simulink model "SimClassic"  (R2017a)
settings: Solver=FixedStepAuto  StartTime=0.0  StopTime=time(end)  FixedStep=0.1  RelTol=1e-3
PostLoadFcn:
  | load Classic_data_2017-11-06_16-06.mat
  | load Trajectory_data_Cux_Visby.rtz2017-11-16_14-55.mat
undefined symbols (not defined in the file): D_psi, D_u, I_psi, I_u, P_psi, P_u, toMpS, toRad, toRPS
settings Model: Creator=c00rts11  LastModifiedBy=c00rts11
settings SolverCC: ZeroCrossAlgorithm=Adaptive

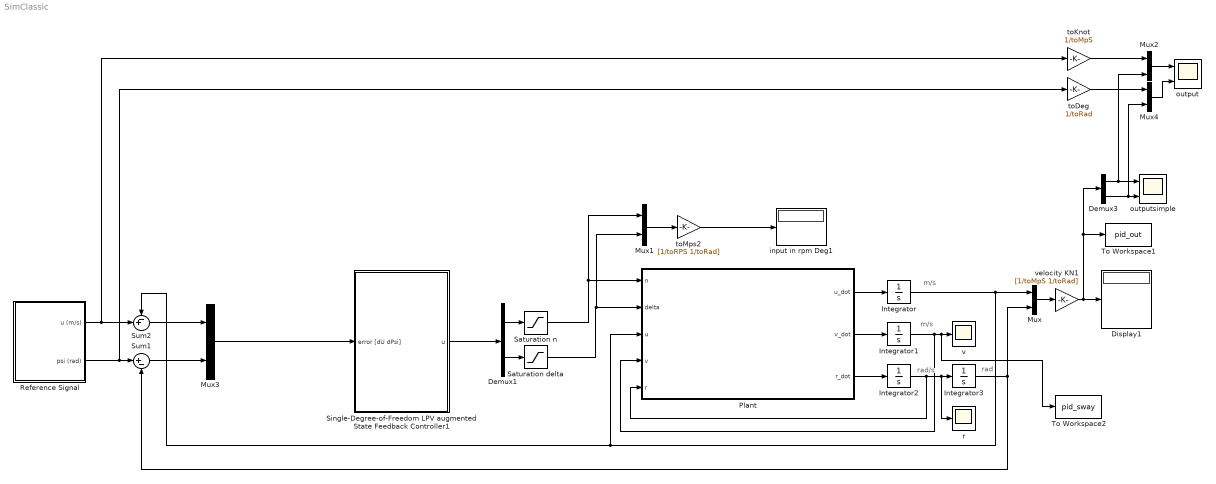
== system SimClassic ==
  note: rad
  note: rad/s
  note: m/s
  note: m/s
  Demux1 : Demux  Outputs=2
  Demux3 : Demux  Outputs=2
  Display1 : Display
  Integrator : Integrator  InitialCondition=0.1*toMpS  UpperSaturationLimit=16*toMpS  LowerSaturationLimit=1e-1*toMpS
  Integrator1 : Integrator  UpperSaturationLimit=0*toMpS  LowerSaturationLimit=-0.001*toMpS
  Integrator2 : Integrator
  Integrator3 : Integrator  WrapState=on  WrappedStateUpperValue=180*toRad  WrappedStateLowerValue=-180*toRad
  Mux{,1..4} (5 alike) : Mux  Inputs=2
  Plant : MATLAB Function  TreatAsAtomicUnit=on
  Reference Signal : Subsystem
  Saturation delta : Saturate  UpperLimit=30*toRad  LowerLimit=-30*toRad  LinearizeAsGain=off
  Saturation n : Saturate  UpperLimit=90*toRPS  LowerLimit=-90*toRPS  LinearizeAsGain=off
  Single-Degree-of-Freedom LPV augmented State Feedback Controller1 : Subsystem
  Sum1 : Sum  Inputs=|+-
  Sum2 : Sum  Inputs=-+|
  To Workspace1 : ToWorkspace  VariableName=pid_out  SaveFormat=Timeseries  SampleTime=-1
  To Workspace2 : ToWorkspace  VariableName=pid_sway  SaveFormat=Timeseries  SampleTime=-1
  input in rpm Deg1 : Display
  output : Scope  NumInputPorts=2
  outputsimple : Scope  NumInputPorts=2
  r : Scope
  toDeg : Gain  Gain=1/toRad
  toKnot : Gain  Gain=1/toMpS
  toMps2 : Gain  Gain=[1/toRPS 1/toRad]
  v : Scope
  velocity KN1 : Gain  Gain=[1/toMpS 1/toRad]
  wires:
  Integrator1/1 -> To Workspace2/1, v/1, Plant/4(v)
  Sum2/1 -> Mux3/1
  Sum1/1 -> Mux3/2
  Saturation n/1 -> Mux1/1, Plant/1(n)
  Plant/2(v_dot) -> Integrator1/1
  Plant/3(r_dot) -> Integrator2/1
  Plant/1(u_dot) -> Integrator/1
  Saturation delta/1 -> Mux1/2, Plant/2(delta)
  toMps2/1 -> input in rpm Deg1/1
  Demux1/2 -> Saturation delta/1
  Integrator/1 -> Mux/1, Sum2/1, Plant/3(u)
  Demux1/1 -> Saturation n/1
  Single-Degree-of-Freedom LPV augmented State Feedback Controller1/1(u) -> Demux1/1
  Mux3/1 -> Single-Degree-of-Freedom LPV augmented State Feedback Controller1/1(error [dU dPsi])
  Integrator2/1 -> Plant/5(r), r/1, Integrator3/1
  Integrator3/1 -> Sum1/2, Mux/2
  Mux1/1 -> toMps2/1
  Mux/1 -> velocity KN1/1
  velocity KN1/1 -> Demux3/1, To Workspace1/1, Display1/1
  Mux4/1 -> output/2
  toDeg/1 -> Mux4/1
  Demux3/1 -> Mux2/2, outputsimple/1
  Demux3/2 -> Mux4/2, outputsimple/2
  Mux2/1 -> output/1
  toKnot/1 -> Mux2/1
  Reference Signal/2(psi (rad)) -> toDeg/1, Sum1/1
  Reference Signal/1(u (m/s)) -> toKnot/1, Sum2/2

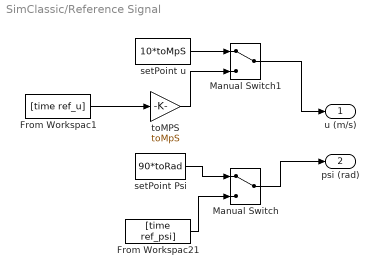
== system SimClassic/Reference Signal ==
  From Workspac1 : FromWorkspace  VariableName=[time ref_u]  SampleTime=0  Interpolate=off  OutputAfterFinalValue=Holding final value
  From Workspac21 : FromWorkspace  VariableName=[time ref_psi]  SampleTime=0  Interpolate=off  OutputAfterFinalValue=Holding final value
  Manual Switch : ManualSwitch
  Manual Switch1 : ManualSwitch
  setPoint Psi : Constant  Value=90*toRad
  setPoint u : Constant  Value=10*toMpS
  toMPS : Gain  Gain=toMpS
  u (m/s) : Outport
  psi (rad) : Outport  Port=2
  wires:
  From Workspac21/1 -> Manual Switch/2
  toMPS/1 -> Manual Switch1/2
  Manual Switch1/1 -> u (m/s)/1
  setPoint u/1 -> Manual Switch1/1
  setPoint Psi/1 -> Manual Switch/1
  Manual Switch/1 -> psi (rad)/1
  From Workspac1/1 -> toMPS/1

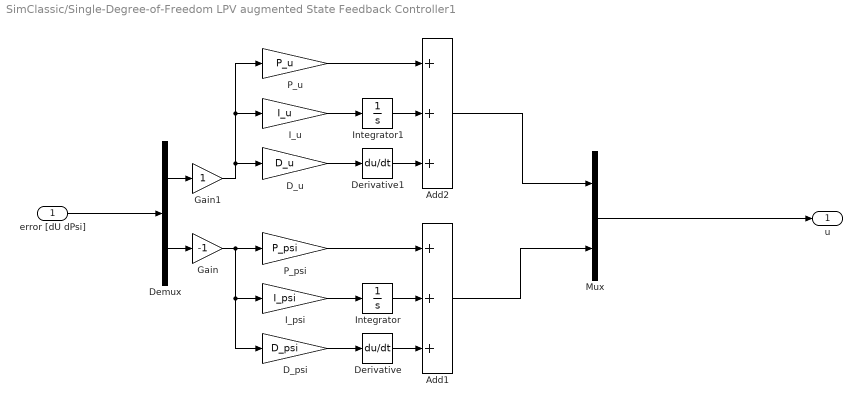
== system SimClassic/Single-Degree-of-Freedom LPV augmented State Feedback Controller1 ==
  error [dU dPsi] : Inport
  Add1 : Sum  Inputs=+++
  Add2 : Sum  Inputs=+++
  D_psi : Gain  Gain=D_psi
  D_u : Gain  Gain=D_u
  Demux : Demux  Outputs=2
  Derivative : Derivative
  Derivative1 : Derivative
  Gain : Gain  Gain=-1
  Gain1 : Gain
  I_psi : Gain  Gain=I_psi
  I_u : Gain  Gain=I_u
  Integrator : Integrator
  Integrator1 : Integrator
  Mux : Mux  Inputs=2
  P_psi : Gain  Gain=P_psi
  P_u : Gain  Gain=P_u
  u : Outport
  wires:
  error [dU dPsi]/1 -> Demux/1
  Demux/2 -> Gain/1
  P_psi/1 -> Add1/1
  Derivative/1 -> Add1/3
  Add1/1 -> Mux/2
  Add2/1 -> Mux/1
  D_u/1 -> Derivative1/1
  P_u/1 -> Add2/1
  I_u/1 -> Integrator1/1
  Integrator1/1 -> Add2/2
  Derivative1/1 -> Add2/3
  Demux/1 -> Gain1/1
  Gain1/1 -> I_u/1, P_u/1, D_u/1
  Gain/1 -> I_psi/1, D_psi/1, P_psi/1
  I_psi/1 -> Integrator/1
  Integrator/1 -> Add1/2
  D_psi/1 -> Derivative/1
  Mux/1 -> u/1

== matlab function SimClassic/Plant ==
  data: n input; delta input; u input; u_dot output; v input; r input; v_dot output; r_dot output
function [u_dot,v_dot,r_dot] = fcn(n,delta,u,v,r)
% n = n/60;
if (u==0)
    u = 1e-5;
end
% Normalization variables
L   =  304.8;          % length of ship (m)
g   =  9.8;            % acceleration of gravity (m/s^2)

% Parameters, hydrodynamic derivatives and main dimensions
% delta_max  = 10;       % max rudder angle      (deg)
% Ddelta_max = 2.33;     % max rudder derivative (deg/s)
% n_max      = 80;       % max shaft velocity    (rpm)

t   =  0.22;
Tm  =  50;
T   =  18.46;

cun =  0.605;  
cnn =  38.2;

Tuu = -0.00695;
Tun = -0.00063;
Tnn =  0.0000354;

m11 =  1.050;          % 1 - Xudot
m22 =  2.020;          % 1 - Yvdot
m33 =  0.1232;         % kz^2 - Nrdot

d11 =  2.020;          % 1 + Xvr
d22 = -0.752;          % Yur - 1
d33 = -0.231;          % Nur - xG 

Xuuz   = -0.0061;   YT     =  0.04;   NT      = -0.02;
Xuu    = -0.0377;   Yvv    = -2.400;  Nvr     = -0.300;
Xvv    =  0.3;      Yuv    = -1.205;  Nuv     = -0.451;   
Xudotz = -0.05;     Yvdotz = -0.387;  Nrdotz  = -0.0045;
Xuuz   = -0.0061;   Yurz   =  0.182;  Nurz    = -0.047;
Xvrz   =  0.387;    Yvvz   = -1.5;    Nvrz    = -0.120;
Xccdd  = -0.093;    Yuvz   =  0;      Nuvz    = -0.241;
Xccbd  =  0.152;    Yccd   =  0.208;  Nccd    = -0.098;
Xvvzz  =  0.0125;   Yccbbd = -2.16;   Nccbbd  =  0.688;
                    Yccbbdz= -0.191;  Nccbbdz =  0.344;

z = T./(50 - T);

% Forces and moments
beta = v/u;
gT   = (1/L*Tuu*u^2 + Tun*u*n + L*Tnn*abs(n)*n);
% C = (cun*u*n + cnn*n^2)*sign(cun*u*n + cnn*n^2);
C = (cun*u*n + cnn*n^2);

gX   = 1/L*(Xuu*u^2 + L*d11*v*r + Xvv*v^2 + Xccdd*C*delta^2 ...
     + Xccbd*C*beta*delta + L*gT*(1-t) + Xuuz*u^2*z ...
     + L*Xvrz*v*r*z + Xvvzz*v^2*z^2);

gY   = 1/L*(Yuv*u*v + Yvv*abs(v)*v + Yccd*C*delta + L*d22*u*r ...
     + Yccbbd*C*abs(beta)*beta*abs(delta) + YT*gT*L ...
     + L*Yurz*u*r*z + Yuvz*u*v*z + Yvvz*abs(v)*v*z  ...
     + Yccbbdz*C*abs(beta)*beta*abs(delta)*z);     

gLN  = Nuv*u*v + L*Nvr*abs(v)*r + Nccd*C*delta +L*d33*u*r ...
     + Nccbbd*C*abs(beta)*beta*abs(delta) + L*NT*gT ...
     + L*Nurz*u*r*z + Nuvz*u*v*z + L*Nvrz*abs(v)*r*z ...
     + Nccbbdz*C*abs(beta)*beta*abs(delta)*z;
 
%  c    = sqrt(cun*u*n + cnn*n^2);
% 
% gX   = 1/L*(Xuu*u^2 + L*d11*v*r + Xvv*v^2 + Xccdd*abs(c)*c*delta^2 ...
%      + Xccbd*abs(c)*c*beta*delta + L*gT*(1-t) + Xuuz*u^2*z ...
%      + L*Xvrz*v*r*z + Xvvzz*v^2*z^2);
% 
% gY   = 1/L*(Yuv*u*v + Yvv*abs(v)*v + Yccd*abs(c)*c*delta + L*d22*u*r ...
%      + Yccbbd*abs(c)*c*abs(beta)*beta*abs(delta) + YT*gT*L ...
%      + L*Yurz*u*r*z + Yuvz*u*v*z + Yvvz*abs(v)*v*z  ...
%      + Yccbbdz*abs(c)*c*abs(beta)*beta*abs(delta)*z);     
% 
% gLN  = Nuv*u*v + L*Nvr*abs(v)*r + Nccd*abs(c)*c*delta +L*d33*u*r ...
%      + Nccbbd*abs(c)*c*abs(beta)*beta*abs(delta) + L*NT*gT ...
%      + L*Nurz*u*r*z + Nuvz*u*v*z + L*Nvrz*abs(v)*r*z ...
%      + Nccbbdz*abs(c)*c*abs(beta)*beta*abs(delta)*z;

m11 = (m11 - Xudotz*z);
m22 = (m22 - Yvdotz*z);
m33 = (m33 - Nrdotz*z);

% Dimensional state derivative
u_dot = gX/m11;
v_dot = gY/m22;
r_dot = gLN/(L^2*m33);
